simulink model "Passo1_5"  (R2016a)
settings: Solver=FixedStepDiscrete  StartTime=0.0  StopTime=Tf  FixedStep=Ts  RelTol=1e-3
values from neighbouring files (symbols this model uses):
  Kx = 0.7682051    [Valid.m]    (also in data_simulation_4.2_MRdamper.mat = 1.064; data_simulation_4.3_MRdamper.mat = 1.31408146066; data_simulation_4.4_MRdamper.mat = 1.31408146066)
  Ts = 0.001    [Valid.m]    (also in data_simulation_4.1_MRdamper.mat = 0.01; data_simulation_4.2_MRdamper.mat = 0.01; data_simulation_4.3_MRdamper.mat; data_simulation_4.4_MRdamper.mat = 0.01)
libraries: powerlib x1
settings Model: Creator=UTFPR  LastModifiedBy=JG
settings DebuggingCC: SFUnexpectedBacktrackingDiag=error  SFNoUnconditionalDefaultTransitionDiag=error
settings GRTTargetCC: TargetLangStandard=C99 (ISO)  GeneratePreprocessorConditionals=Use local settings
settings ConfigComp: CovMetricSettings=dwe  CovHtmlReporting=off  CovSaveCumulativeToWorkspaceVar=off  CovSaveSingleToWorkspaceVar=off  CovExternalEMLEnable=on

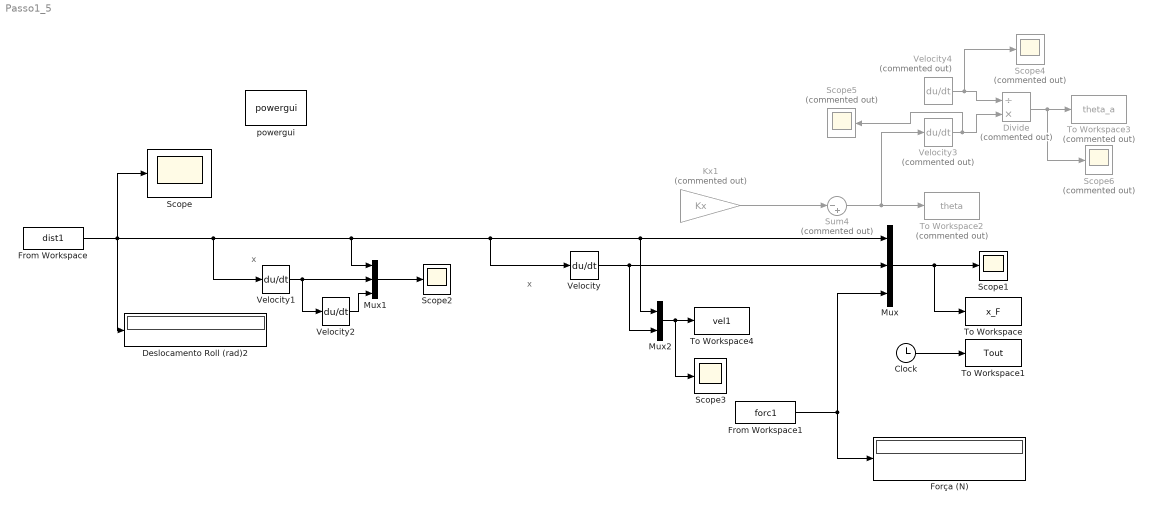
== system Passo1_5 ==
  note: x
  note: x
  Clock : Clock
  Deslocamento Roll (rad)2 : Display
  Divide : Product  Commented=on  Inputs=/*  SampleTime=Ts
  Força (N) : Display
  From Workspace : FromWorkspace  VariableName=dist1  OutDataTypeStr=double  SampleTime=Ts
  From Workspace1 : FromWorkspace  VariableName=forc1
  Kx1 : Gain  Commented=on  Gain=Kx  SampleTime=Ts
  Mux : Mux  Inputs=3
  Mux1 : Mux  Inputs=3
  Mux2 : Mux  Inputs=2
  Scope{,1..3} (4 alike) : Scope
  Scope4 : Scope  Commented=on
  Scope5 : Scope  Commented=on
  Scope6 : Scope  Commented=on
  Sum4 : Sum  Commented=on  Inputs=|-+  SampleTime=Ts
  To Workspace : ToWorkspace  VariableName=x_F  SampleTime=Ts
  To Workspace1 : ToWorkspace  VariableName=Tout  SampleTime=Ts
  To Workspace2 : ToWorkspace  Commented=on  VariableName=theta  SampleTime=Ts
  To Workspace3 : ToWorkspace  Commented=on  VariableName=theta_a  SampleTime=Ts
  To Workspace4 : ToWorkspace  VariableName=vel1  SampleTime=Ts
  Velocity : Derivative
  Velocity1 : Derivative
  Velocity2 : Derivative
  Velocity3 : Derivative  Commented=on
  Velocity4 : Derivative  Commented=on
  powergui : powerlib/powergui  Priority=1  SimulationMode=Discrete  SampleTime=Ts  frequency=60  Iterations=50  frequencyindice=60  Pbase=100e6  ErrMax=1e-4  UnitsV=kV  UnitsW=MW  buscounter=0  FunctionMessages=off  echomessages=off  EnableUseOfTLC=off  CurrentSourceSwitches=off  DisableSnubberDevices=off  DisableRonSwitches=off  DisableVfSwitches=off  DisplayEquations=off  SolverType=Tustin  Interpol=off  ExternalGateDelay=off  methode=off  Ts=10  x0status=blocks  SPID=off  SwTol=0  HookPort=off  RestoreLinks=warning  ResistiveCurrentMeasurement=off  Frange=[0:2:500]  Ylog=off  Xlog=on  ShowGrid=off  save=off  variable=ZData  structure=0  ZoomFFT=off  StartTime=0.0  cycles=1  DisplayStyle=1  fundamental=60  FreqAxis=off  MaxFrequency=1000  frequencyindicesteady=1  RmsSteady=1  display=off
  wires:
  Velocity/1 -> Mux2/2, Mux/2
  Mux/1 -> To Workspace/1, Scope1/1
  Mux1/1 -> Scope2/1
  Velocity1/1 -> Velocity2/1, Mux1/2
  Clock/1 -> To Workspace1/1
  From Workspace/1 -> Scope/1, Deslocamento Roll (rad)2/1, Velocity1/1, Mux1/1, Velocity/1, Mux2/1, Mux/1
  Velocity2/1 -> Mux1/3
  Kx1/1 -> Sum4/1
  Sum4/1 -> Velocity3/1, To Workspace2/1
  Velocity4/1 -> Scope4/1, Divide/1
  Velocity3/1 -> Scope5/1, Divide/2
  Divide/1 -> Scope6/1, To Workspace3/1
  From Workspace1/1 -> Força (N)/1, Mux/3
  Mux2/1 -> Scope3/1, To Workspace4/1
